simulink model "VisionModel_v16"  (Simulink 7.6)
settings: Solver=FixedStepDiscrete  StartTime=0.0  StopTime=0  RelTol=1e-3
values from neighbouring files (symbols this model uses):
  Buoy_Max_Eccentricity = 1.2    [VisionConstants.m]
  Buoy_Max_Extent = 0.9    [VisionConstants.m]
  Buoy_Min_Eccentricity = 0    [VisionConstants.m]
  Buoy_Min_Extent = 0.1    [VisionConstants.m]
  Down_Camera_Dimensions = [120 160]    [VisionConstants.m]
  Forward_Camera_Dimensions = [160 120]    [VisionConstants.m]
undefined symbols (not defined in the file or in its folder): Forward_Fov, Rec, SDTV
libraries: vipconversions x8, vipgeotforms x6, viptextngfix x6, viptransforms x4, vipanalysis x3
(part 3 of 4)

== matlab function validation_gate/Identify Validation Gate ==
  data: hough_table input double; target_y output double; target_z output double; target_yaw output double; gate_found output double; theta_in input double; rho_in input double; target_height input double; gate_aspect_ratio input double; Forward_Camera_Dimensions input double; Forward_Fov input double; rho_gate output double; theta_gate output double
function [target_y, target_z, target_yaw, gate_found, rho_gate, theta_gate] = validation_gate(hough_table, theta_in, rho_in, target_height, gate_aspect_ratio, Forward_Camera_Dimensions, Forward_Fov)
%#eml



% This function attempts to identfiy the validation gate, and returns
%   targeting information, and a true/false gate_found parameter.
%
% 5-29-11
%
% Input
%
%   target_height = fraction of goal post height to aim AUV at
%   gate_aspect_ratio = used to infer unknown points with little extra
%     processing (height/width of large goalpost-shape)
%
% Output
%
% Notes:
%   The hough_table is destroyed in this function (acceptable if
%     hough_table is not an output)
%   Process:
%     1. Identify primary, relatively "long" lines
%     2. 


%% Initialize
% Only the (max_num_lines) with the most votes will be considered as
%   candidates for the validation gate
max_num_lines = 200;
[rho_length, theta_length] = size(hough_table);
%rows = Forward_Camera_Dimensions(1);
%cols = Forward_Camera_Dimensions(2);
%rows = 120;
%cols = 160;
rows = 160;
cols = 120;


% eps_rho must be at least as big as the gate leg diameter (units of
%   pixels)
eps_rho = .1*max(rows,cols);
% eps_theta is used to distinguish lines as "horizontal" or "vertical";
%   units are radians
eps_theta = 10*pi/180;


% These vectors contain the final three lines that compose the validation gate
rho_gate = zeros(1,3);
theta_gate = zeros(1,3);

% These vectors contain intermediate line information; as lines are
%   eliminated from these vectors, their values are set to zero
rho = zeros(1,max_num_lines);
theta = zeros(1,max_num_lines);





% Identify the most popular max_num_lines lines
i_index = ones(1,max_num_lines);
j_index = ones(1,max_num_lines);

m = 1;
while( m <= max_num_lines )
    
    max_votes = 0;
    for i = 1:rho_length
        for j = 1:theta_length
            if( hough_table(i,j) > max_votes )
                i_index(m) = i;
                j_index(m) = j;
                max_votes = hough_table(i,j);
            end
        end
    end
    
    rho(m) = rho_in(i_index(m));
    theta(m) = theta_in(j_index(m));
    hough_table(i_index(m),j_index(m)) = 0;
    m = m + 1;
    
end


% Effectively generate a small Hough table which contains only values of
%   interest for the validation gate application

rbinv = [0:(2*eps_rho):max(rows, cols)];  % Rho bins for vertical lines
nbinsv = length(rbinv);  % Number of rho bins for vertical lines
ravgv = zeros(1,nbinsv);  % Average rho values for each bin (note that the average value will generally differ slightly than the bin value)
tavgv = zeros(1,nbinsv);  % Average theta values for each bin
vbinv = zeros(1,nbinsv);  % Votes bins for vertical lines

rbinh = [0:(2*eps_rho):max(rows, cols)];
nbinsh = length(rbinh);
ravgh = zeros(1,nbinsh);
tavgh = zeros(1,nbinsh);
vbinh = zeros(1,nbinsh);

% Allow vertical lines along the left side of the image
rbinv(1) = 1;
rbinh(1) = 1;

for i = 1:max_num_lines
    
    % Consider only lines that are either vertical or horizontal, within
    %   tolerance
    condition1 = ( abs(theta(i) - pi/2) <= eps_theta || abs(theta(i) + pi/2) <= eps_theta );  % Horizontal line
    condition2 = ( abs(theta(i) - 0) <= eps_theta );  % Vertical line
    
    if(condition2 && ~( rho(i) == 0 && theta(i) == 0 ))  % Analyze vertical lines (ignore lines exactly along the left side of the image)
        
        for b = 1:nbinsv
            
            % Place each rho value into a bin
            if( abs(rho(i) - rbinv(b)) <= eps_rho )
                ravgv(b) = ravgv(b) + rho(i);
                tavgv(b) = tavgv(b) + theta(i);
                vbinv(b) = vbinv(b) + 1;
                break;
            end
            
        end
        
    elseif(condition1)  % Analyze horizontal lines
        
        if( theta(i) < 0 )
            theta(i) = theta(i) + pi;
            rho(i) = -rho(i);
        end
        
        for b = 1:nbinsh
            
            % Place each rho value into a bin
            if( abs(rho(i) - rbinh(b)) <= eps_rho )
                ravgh(b) = ravgh(b) + rho(i);
                tavgh(b) = tavgh(b) + theta(i);
                vbinh(b) = vbinh(b) + 1;
                break;
            end
            
        end
        
    end
end

% Average the values in ravg and tavg for horizontal and vertical lines
for b = 1:nbinsv
    if( vbinv(b) == 0 )
        ravgv(b) = 0;
        tavgv(b) = 0;
    else
        ravgv(b) = ravgv(b)./vbinv(b);
        tavgv(b) = tavgv(b)./vbinv(b);
    end
end
for b = 1:nbinsh
    if( vbinh(b) == 0 )
        ravgh(b) = 0;
        tavgh(b) = 0;
    else
        ravgh(b) = ravgh(b)./vbinh(b);
        tavgh(b) = tavgh(b)./vbinh(b);
    end
end


%% Extract three lines that fit the criteria for being the validation gate
rmin = 10000;
rmax = -10000;
for b = 1:nbinsv
    
    % Extract the left-most vertical line
    if( ravgv(b) < rmin && ravgv(b) ~= 0 )
        rmin = ravgv(b);
        rho_gate(1) = ravgv(b);
        theta_gate(1) = tavgv(b);
    end
    
    % Extract the right-most vertical line
    if( ravgv(b) > rmax && ravgv(b) ~= 0 )
        rmax = ravgv(b);
        rho_gate(3) = ravgv(b);
        theta_gate(3) = tavgv(b);
    end
    
end

% Check that the distance between the vertical lines is much greater than
%   the minimum expected distance, eps_rho
if( abs(rho_gate(3) - rho_gate(1)) < 2*eps_rho )
    rho_gate(1) = 0;
    rho_gate(3) = 0;
    theta_gate(1) = 0;
    theta_gate(3) = 0;
end

%rmin = 10000;
vmax = 0;
for b = 1:nbinsh
    
    % Extract the horizontal line with the most votes
    if( vbinh(b) > vmax && ravgh(b) ~= 0 )
        vmax = vbinh(b);
        rho_gate(2) = ravgh(b);
        theta_gate(2) = tavgh(b);
    end
    
%    % Extract the horizontal line that is highest up in the image
%    if( ravgh(b) < rmin && ravgh(b) ~= 0 )
%        rmin = ravgh(b);
%        rho_gate(2) = ravgh(b);
%        theta_gate(2) = tavgh(b);
%    end
end


%% Compute targeting information
% Compute intersections
r1 = (  ( rho_gate(1)/cos(theta_gate(1)) ) - ( rho_gate(2)/cos(theta_gate(2)) )  )*(  1/( tan(theta_gate(1)) - tan(theta_gate(2)) )  );
c1 = ( 1/cos(theta_gate(1)) )*( rho_gate(1) - r1*sin(theta_gate(1)) );

r3 = (  ( rho_gate(2)/cos(theta_gate(2)) ) - ( rho_gate(3)/cos(theta_gate(3)) )  )*(  1/( tan(theta_gate(2)) - tan(theta_gate(3)) )  );
c3 = ( 1/cos(theta_gate(2)) )*( rho_gate(2) - r3*sin(theta_gate(2)) );

r2 = (r1 + r3)/2;
c2 = (c1 + c3)/2;

% Compute gate width
w = sqrt( (r3 - r1)^2 + (c3 - c1)^2 );

% Form unit vector pointing downward, parallel to gate posts
tavg = ( theta_gate(1) + (theta_gate(2) - pi/2) + theta_gate(3) )/3;
u = [1 tan(tavg)];
u = u./norm(u);

% Compute target location
th = target_height*gate_aspect_ratio*w;
r_t = r2 + th*u(1);
c_t = c2 + th*u(2);

% Determine if a gate is present (very simple, potentially inaccurate)
if( sum( (rho_gate == 0) + (theta_gate == 0) ) > 0 )
    
    gate_found = 0;
    target_z = 0;
    target_y = 0;
    target_yaw = 0;
    
else
    
    gate_found = 1;
    
    % Transform target r, c to global coordinate system
    target_z = r_t - floor(rows/2);
    target_y = c_t - floor(cols/2);
    target_yaw = Forward_Fov*(target_y/cols);
    
end


return

== matlab function validation_gate/If Action Subsystem/Transform Coordinates3 ==
  data: which_camera input double; x_in input double; y_in input double; z_in input double; Camera_Dimensions input double; points output double
function points = transform_G2L(which_camera, x_in, y_in, z_in, Camera_Dimensions)
% This function, "transform Global to Local coordinates," transforms
%   global coordinates that are sent to the controller into local
%   coordinates that can be displayed over images.
%
% 5-29-11
%
% Input
%   x_in, y_in, z_in = vectors of points in global (vehicle-centered)
%     coordinate system
%   bw_image_in = a 2-D array of pixel values (used only to extract image
%     size)
%   which_camera = selects which camera for relative coordinates
%                = 0 -> Forward camera
%                = 1 -> Down camera
%
% Output
%   r_out, c_out = row, column pairs in local coordinate system

rows = Camera_Dimensions(1);
cols = Camera_Dimensions(2);
if( which_camera == 0 )
    points = [z_in + floor(rows/2);
              y_in + floor(cols/2)];
else
    points = [floor(rows/2) - x_in;
              y_in + floor(cols/2)];
end


return

== matlab function L_detector/If Action Subsystem/Transform Coordinates3 ==
  data: which_camera input double; x_in input double; y_in input double; z_in input double; Camera_Dimensions input double; points output double
function points = transform_G2L(which_camera, x_in, y_in, z_in, Camera_Dimensions)
% This function, "transform Global to Local coordinates," transforms
%   global coordinates that are sent to the controller into local
%   coordinates that can be displayed over images.
%
% 5-29-11
%
% Input
%   x_in, y_in, z_in = vectors of points in global (vehicle-centered)
%     coordinate system
%   bw_image_in = a 2-D array of pixel values (used only to extract image
%     size)
%   which_camera = selects which camera for relative coordinates
%                = 0 -> Forward camera
%                = 1 -> Down camera
%
% Output
%   r_out, c_out = row, column pairs in local coordinate system

rows = Camera_Dimensions(1);
cols = Camera_Dimensions(2);
if( which_camera == 0 )
    points = [z_in + floor(rows/2);
              y_in + floor(cols/2)];
else
    points = [floor(rows/2) - x_in;
              y_in + floor(cols/2)];
end


return

== matlab function Blob_Analysis1/Blob Extraction ==
  data: LabelMatrix input double; num_colors input double; ref_colors input double; blob_hues output double; blob_area output double; blob_centroids output double; blob_bbox output double; blob_major_axis output double; blob_minor_axis output double; blob_orientation output double; blob_eccentricity output double; blob_extent output double; blob_count output double; blob_color output double; bw_image output double; ColorFilter_in input double
function [blob_hues, blob_area, blob_centroids, blob_bbox, blob_major_axis, blob_minor_axis, blob_orientation, blob_eccentricity, blob_extent, blob_count, blob_color, bw_image] = GetBlobInfo(LabelMatrix, num_colors, ref_colors, ColorFilter_in)
% This function calculates blob information for each color component after
%   iterative segmentation


% Output
%   blob_color = 1xN vector of color indices (global color scheme)


% Initialize


%{
a_range =[0     0     0    25   127    70    50;
     0     0     0   127   -18   -40   -82];


b_range =[0     0     0     0    30   -13   -40;
     0     0     0    56   -10    30     9];
%}

%ColorFilter = ColorFilter_in;



cf = [0 1 0 0 0 0 0;
0     0     0    25   127    70    50;
0     0     0   127   -18   -40   -82;
0     0     0     0    30   -13   -40;
0     0     0    56   -10    30     9];

ColorFilter = ColorFilter_in(:,1);
a_range = cf(2:3,:);
b_range = cf(4:5,:);

max_num_blobs = 50;
min_blob_area = 5;

[rows, cols] = size(LabelMatrix);
image_area = rows*cols;
LogicMatrix = false(rows,cols);
bw_image = zeros(rows,cols);

blob_hues = zeros(3,max_num_blobs);
blob_area = -1.*ones(1,max_num_blobs);
blob_bbox = zeros(4,max_num_blobs);
blob_major_axis = zeros(1,max_num_blobs);
blob_minor_axis = zeros(1,max_num_blobs);
blob_centroids = zeros(2,max_num_blobs);
blob_eccentricity = zeros(1,max_num_blobs);
blob_extent = zeros(1,max_num_blobs);
blob_orientation = zeros(1,max_num_blobs);
blob_count = 0;

blob_color = zeros(1,max_num_blobs);

max_num_col_filter = length(ColorFilter);
num_col_filter = sum(ColorFilter);

area_thresh = .1;


% Determine L_white and L_black as needed
find_white = 0;
find_black = 0;
L_white = 101;
L_black = -1;
color_areas = zeros(1,size(ref_colors,1));

if(ColorFilter(1) + ColorFilter(2) > 0)
    for row = 1:rows
        for col = 1:cols
            color_areas(LabelMatrix(row,col)) = color_areas(LabelMatrix(row,col)) + 1;
        end
    end
end

if(ColorFilter(1) == 1)
    
    % Determine the brightest colors, but allow a maximum area
    %   ratio of the image to be "white"
    find_white = 1;
    
    positive_area = 0;
    for n = 1:num_colors
        
        maxL = -1;
        k_max = -1;
        for k = 1:num_colors
            L = ref_colors(k,1);
            if(L > maxL && L < L_white)
                maxL = L;
                k_max = k;
            end
        end
        
        positive_area = positive_area + color_areas(k_max);
        if(positive_area/image_area >= area_thresh && n > 1)
            break;
        end
        
        L_white = maxL;
        
    end
end

if(ColorFilter(2) == 1)
    
    % Determine the darkest colors, but allow a maximum area
    %   ratio of the image to be "black"
    find_black = 1;
    
    for row = 1:rows
        for col = 1:cols
            color_areas(LabelMatrix(row,col)) = color_areas(LabelMatrix(row,col)) + 1;
        end
    end
    
    positive_area = 0;
    for n = 1:num_colors
        
        minL = 101;
        k_min = -1;
        for k = 1:num_colors
            L = ref_colors(k,1);
            if(L < minL && L > L_black)
                minL = L;
                k_min = k;
            end
        end
        
        positive_area = positive_area + color_areas(k_min);
        if(positive_area/image_area >= area_thresh && n > 1)
            break;
        end
        
        L_black = minL;
        
    end
end


% Input hblob, a matrix containing [Area, blob_centroids, Eccentricity] for each
% identified blob
persistent hblob
if isempty(hblob)
    hblob = video.BlobAnalysis('AreaOutputPort',true,'CentroidOutputPort',true,...
        'BoundingBoxOutputPort',true,'MajorAxisLengthOutputPort',true,'MinorAxisLengthOutputPort',true,...
        'OrientationOutputPort',true,...
        'EccentricityOutputPort',true,'ExtentOutputPort',true,'NumBlobsOutputPort',true,...
        'MinimumBlobAreaSource','Property','MinimumBlobArea', min_blob_area);
end


% Calculate geometric information about the blobs
%
% LogicMatrix is a binary version of LabelMatrix, with ones at all
%   locations for which color values are k, and zeros everywhere else
%
% Explanation
%   condition1 == 1 causes the k'th color to be analyzed by blob analysis,
%     as well as be included in the black-and-white image
%   condition1 == 0 disallows both of these items and simply ignores color
%     k
%   condition0 == 1 ensures that condition1 is true for all k
%   condition0 == 0 enforces a filter which allows only the colors
%     specified in the ColorFilter vector
condition0 = (num_col_filter == 0);
current_color = 0;
for k = 1:num_colors
    
    % Decide whether or not to perform blob analysis
    condition1 = 0;
    if(condition0)
        condition1 = 1;
    else
        a = ref_colors(k, 2);
        b = ref_colors(k, 3);
        for i = 1:max_num_col_filter
            
            % Skip colors that have not been specified
            if(ColorFilter(i) == 0)
                continue;
            end
            
            if( find_white == 1 && ref_colors(k,1) >= L_white)  % Handle "white" differently than other colors
                condition1 = 1;
                current_color = 1;
                break;
            elseif( find_black == 1 && ref_colors(k,1) <= L_black)  % Handle "black" differently than other colors
                condition1 = 1;
                current_color = 2;
                break;
            elseif( a >= a_range(1,i) && a <= a_range(2,i) && b >= b_range(1,i) && b <= b_range(2,i) )
                condition1 = 1;
                current_color = i;
                break;
            end
            
        end
    end
    
    % Blob analysis
    if( condition1 == 1 )
        
        for i = 1:rows
            for j = 1:cols
                if(LabelMatrix(i,j) ~= k)
                    LogicMatrix(i,j) = false;
                else
                    LogicMatrix(i,j) = true;
                    bw_image(i,j) = 1;
                end
            end
        end

        [TArea,TCentroid,TBBox,TMajorAxis,TMinorAxis,TOrientation,TEccent,TExtent,TNumBlobs] = step(hblob,LogicMatrix);

        for i = 1:TNumBlobs
            if(blob_count + TNumBlobs <= max_num_blobs)

                blob_centroids(1,blob_count+i) = TCentroid(1,i);
                blob_centroids(2,blob_count+i) = TCentroid(2,i);

                ii = round(blob_centroids(1,blob_count+i));
                jj = round(blob_centroids(2,blob_count+i));

                blob_hues(1,blob_count+i) = ref_colors( LabelMatrix(ii,jj), 1 );
                blob_hues(2,blob_count+i) = ref_colors( LabelMatrix(ii,jj), 2 );
                blob_hues(3,blob_count+i) = ref_colors( LabelMatrix(ii,jj), 3 );

                blob_area(blob_count+i) = TArea(i);
                blob_bbox(blob_count+i) = TBBox(i);
                blob_major_axis(blob_count+i) = TMajorAxis(i);
                blob_minor_axis(blob_count+i) = TMinorAxis(i);
                blob_eccentricity(blob_count+i) = TEccent(i);
                blob_extent(blob_count+i) = TExtent(i);
                blob_orientation(blob_count+i) = TOrientation(i);
                
                blob_color(blob_count+i) = current_color;

            end
        end

        blob_count = blob_count + double(TNumBlobs);

    end
    
end


return

== matlab function Blob_Analysis1/IterativeSegmentation/Low Pass Filter/Low Pass Filter ==
  data: I input double; Iout output double
function Iout = GaussianBlurr(I)
% This function calculates the gaussian blur of an intensity image

sigma = sqrt(2);

Grows = 3;    % Gaussian matrix rows
Gcols = 3;    % Gaussian matrix columns

[Irows Icols] = size(I);

Iout = double(zeros(Irows,Icols));

Trows = Irows - Grows + 1;
Tcols = Icols - Gcols + 1;
Itemp = double(zeros(Trows,Tcols));

G = zeros(Grows,Gcols);

FirstRow = ceil(-Grows/2);
LastRow = floor(Grows/2);
FirstCol = ceil(-Gcols/2);
LastCol = floor(Gcols/2);
Gsum = 0;
for i=FirstRow:LastRow
    for j = FirstCol:LastCol
        G(i-FirstRow+1,j-FirstCol+1) = exp(-(j*j+i*i)/(2*sigma*sigma));
        Gsum = Gsum + G(i-FirstRow+1,j-FirstCol+1);
    end
end

G = G./Gsum;

Itemp = conv2(double(I),double(G),'valid');

% reflect boundaries to keep image the same size
% top
Iout((1:LastRow),(LastCol+1:Icols-LastCol)) = Itemp((1:LastRow),(1:Tcols));
% bottom
Iout((Irows-LastRow+1:Irows),(LastCol+1:Icols-LastCol)) = Itemp((Trows-LastRow+1:Trows),(1:Tcols));
% left
Iout((1+LastRow:Irows-LastRow),(1:LastCol)) = Itemp((1:Trows),(1:LastCol));
% right
Iout((1+LastRow:Irows-LastRow),(Icols-LastCol+1:Icols)) = Itemp((1:Trows),(Tcols-LastCol+1:Tcols));
% center
Iout((1+LastRow:Irows-LastRow),(1+LastCol:Icols-LastCol)) = Itemp;
% top left corner
Iout(1:LastRow,1:LastCol) = Itemp(1:LastRow,1:LastCol);
% top right corner
Iout(1:LastRow,Icols-LastCol:Icols) = Itemp(1:LastRow,Tcols-LastCol:Tcols);
% bottom left corner
Iout(Irows-LastRow:Irows,1:LastCol) = Itemp(Trows-LastRow:Trows,1:LastCol);
% bottom right corner
Iout(Irows-LastRow:Irows,Icols-LastCol:Icols) = Itemp(Trows-LastRow:Trows,Tcols-LastCol:Tcols);

return

== matlab function Blob_Analysis1/IterativeSegmentation/Low Pass Filter/Low Pass Filter1 ==
  data: I input double; Iout output double
function Iout = GaussianBlurr(I)
% This function calculates the gaussian blur of an intensity image

sigma = sqrt(2);

Grows = 3;    % Gaussian matrix rows
Gcols = 3;    % Gaussian matrix columns

[Irows Icols] = size(I);

Iout = double(zeros(Irows,Icols));

Trows = Irows - Grows + 1;
Tcols = Icols - Gcols + 1;
Itemp = double(zeros(Trows,Tcols));

G = zeros(Grows,Gcols);

FirstRow = ceil(-Grows/2);
LastRow = floor(Grows/2);
FirstCol = ceil(-Gcols/2);
LastCol = floor(Gcols/2);
Gsum = 0;
for i=FirstRow:LastRow
    for j = FirstCol:LastCol
        G(i-FirstRow+1,j-FirstCol+1) = exp(-(j*j+i*i)/(2*sigma*sigma));
        Gsum = Gsum + G(i-FirstRow+1,j-FirstCol+1);
    end
end

G = G./Gsum;

Itemp = conv2(double(I),double(G),'valid');

% reflect boundaries to keep image the same size
% top
Iout((1:LastRow),(LastCol+1:Icols-LastCol)) = Itemp((1:LastRow),(1:Tcols));
% bottom
Iout((Irows-LastRow+1:Irows),(LastCol+1:Icols-LastCol)) = Itemp((Trows-LastRow+1:Trows),(1:Tcols));
% left
Iout((1+LastRow:Irows-LastRow),(1:LastCol)) = Itemp((1:Trows),(1:LastCol));
% right
Iout((1+LastRow:Irows-LastRow),(Icols-LastCol+1:Icols)) = Itemp((1:Trows),(Tcols-LastCol+1:Tcols));
% center
Iout((1+LastRow:Irows-LastRow),(1+LastCol:Icols-LastCol)) = Itemp;
% top left corner
Iout(1:LastRow,1:LastCol) = Itemp(1:LastRow,1:LastCol);
% top right corner
Iout(1:LastRow,Icols-LastCol:Icols) = Itemp(1:LastRow,Tcols-LastCol:Tcols);
% bottom left corner
Iout(Irows-LastRow:Irows,1:LastCol) = Itemp(Trows-LastRow:Trows,1:LastCol);
% bottom right corner
Iout(Irows-LastRow:Irows,Icols-LastCol:Icols) = Itemp(Trows-LastRow:Trows,Tcols-LastCol:Tcols);

return

== matlab function Blob_Analysis1/IterativeSegmentation/Low Pass Filter/Low Pass Filter2 ==
  data: I input double; Iout output double
function Iout = GaussianBlurr(I)
% This function calculates the gaussian blur of an intensity image

sigma = sqrt(2);

Grows = 3;    % Gaussian matrix rows
Gcols = 3;    % Gaussian matrix columns

[Irows Icols] = size(I);

Iout = double(zeros(Irows,Icols));

Trows = Irows - Grows + 1;
Tcols = Icols - Gcols + 1;
Itemp = double(zeros(Trows,Tcols));

G = zeros(Grows,Gcols);

FirstRow = ceil(-Grows/2);
LastRow = floor(Grows/2);
FirstCol = ceil(-Gcols/2);
LastCol = floor(Gcols/2);
Gsum = 0;
for i=FirstRow:LastRow
    for j = FirstCol:LastCol
        G(i-FirstRow+1,j-FirstCol+1) = exp(-(j*j+i*i)/(2*sigma*sigma));
        Gsum = Gsum + G(i-FirstRow+1,j-FirstCol+1);
    end
end

G = G./Gsum;

Itemp = conv2(double(I),double(G),'valid');

% reflect boundaries to keep image the same size
% top
Iout((1:LastRow),(LastCol+1:Icols-LastCol)) = Itemp((1:LastRow),(1:Tcols));
% bottom
Iout((Irows-LastRow+1:Irows),(LastCol+1:Icols-LastCol)) = Itemp((Trows-LastRow+1:Trows),(1:Tcols));
% left
Iout((1+LastRow:Irows-LastRow),(1:LastCol)) = Itemp((1:Trows),(1:LastCol));
% right
Iout((1+LastRow:Irows-LastRow),(Icols-LastCol+1:Icols)) = Itemp((1:Trows),(Tcols-LastCol+1:Tcols));
% center
Iout((1+LastRow:Irows-LastRow),(1+LastCol:Icols-LastCol)) = Itemp;
% top left corner
Iout(1:LastRow,1:LastCol) = Itemp(1:LastRow,1:LastCol);
% top right corner
Iout(1:LastRow,Icols-LastCol:Icols) = Itemp(1:LastRow,Tcols-LastCol:Tcols);
% bottom left corner
Iout(Irows-LastRow:Irows,1:LastCol) = Itemp(Trows-LastRow:Trows,1:LastCol);
% bottom right corner
Iout(Irows-LastRow:Irows,Icols-LastCol:Icols) = Itemp(Trows-LastRow:Trows,Tcols-LastCol:Tcols);

return

== matlab function Blob_Analysis1/IterativeSegmentation/Segmentation/LabSegmentation ==
  data: L input double; LabelMatrix output double; a input double; b input double; ref_colors input double; num_colors input double
function LabelMatrix  = LabSegmentation(L,a,b,ref_colors,num_colors)
% This function generates the label matrix

[rows cols] = size(L);
LabelMatrix = zeros(rows,cols);

for i = 1:rows
    for j = 1:cols
        min_dist = 1000;
        index = 1;
        for k = 1:num_colors
            dist = sqrt((ref_colors(k,1) - L(i,j))^2 + (ref_colors(k,2) - a(i,j))^2 + (ref_colors(k,3) - b(i,j))^2);
            if(dist < min_dist)
                min_dist = double(dist);
                index = k;
            end
        end
        LabelMatrix(i,j) = index;
    end
end


return

== matlab function Blob_Analysis1/IterativeSegmentation/Segmentation/Reference Color Selection ==
  data: L input double; ref_colors output double; a input double; b input double; num_colors output double; Dist_Thresh input double
function [ref_colors, num_colors] = Segmentation(L,a,b,Dist_Thresh)
% This function tries segmentation by adding new reference colors everytime
% a pixel is found with a distance greater than a certain amount from
% every other reference color

[rows cols] = size(L);

Dist_Threshold = Dist_Thresh;% L = 0 to 100, a = -100 to 100, b = -100 to 100
                    % max dist = 300 -> 60/300 is 20%
x = 1;  % coefficients determining distance calculation
y = 1.5;
z = 1.5;

max_num_colors = 50;
ref_colors = zeros(max_num_colors,3);   % At most 50 different reference colors
LabelMatrix = zeros(rows,cols);
num_colors = 1;

center_row = floor(rows/2);
center_col = floor(cols/2);

% Define first reference color to be colr
ref_colors(1,:) = [L(center_row,center_col) a(center_row,center_col) b(center_row,center_col)];

flag = 0;
i = 1;
j = 1;
while(i <= rows)        % perform initial segmentation
    while(i <= rows && flag == 0)
        while(j <= cols && flag == 0)
            k = 1;
            min_dist = 1000;
            index = 1;
            while(k <= num_colors)
                dist = sqrt(x*(ref_colors(k,1) - L(i,j))^2 + y*(ref_colors(k,2) - a(i,j))^2 + z*(ref_colors(k,3) - b(i,j))^2);
                if(min_dist > dist)
                    min_dist = double(dist);
                    index = k;
                end
                k = k + 1;
            end
            if(j == 117)
                cow = 1;
            end
            if(min_dist > Dist_Threshold && num_colors < max_num_colors)
                ref_colors(num_colors+1,:) = [L(i,j) a(i,j) b(i,j)];
                num_colors = num_colors + 1;
                flag = 1;
                i = 0;
                j = 0;
            else
                LabelMatrix(i,j) = index;
            end
            j = j + 1;
        end
        j = 1;
        i = i + 1;
    end
    flag = 0;
end

% Go through image once more to get more accurate values for the different regions
ref_color_L_avg = zeros(50,1);
ref_color_a_avg = zeros(50,1);
ref_color_b_avg = zeros(50,1);
color_count = zeros(50,1);
for i = 1:rows
    for j = 1:cols
        index = LabelMatrix(i,j);
        ref_color_L_avg(index) = ref_color_L_avg(index) + L(i,j);
        ref_color_a_avg(index) = ref_color_a_avg(index) + a(i,j);
        ref_color_b_avg(index) = ref_color_b_avg(index) + b(i,j);
        color_count(index) = color_count(index) + 1;
    end
end
ref_color_L_avg = ref_color_L_avg ./ color_count;
ref_color_a_avg = ref_color_a_avg ./ color_count;
ref_color_b_avg = ref_color_b_avg ./ color_count;

for i = 1:num_colors
    ref_colors(i,1) = ref_color_L_avg(i);
    ref_colors(i,2) = ref_color_a_avg(i);
    ref_colors(i,3) = ref_color_b_avg(i);
end

return

== matlab function Blob_Analysis1/Segmented Image/Display Image ==
  data: LabelMatrix input double; ref_colors input double; L output double; a output double; b output double
function [L, a, b] = Display_Image(LabelMatrix, ref_colors)


% Initialize
[rows,cols] = size(LabelMatrix);
L = zeros(rows,cols);
a = zeros(rows,cols);
b = zeros(rows,cols);


% Allow only colors in specified range
for r = 1:rows
    for c = 1:cols
        
        L(r,c) = ref_colors(LabelMatrix(r,c), 1);
        a(r,c) = ref_colors(LabelMatrix(r,c), 2);
        b(r,c) = ref_colors(LabelMatrix(r,c), 3);
        
    end
end


return

== matlab function path_detector/Identify Path Elements ==
  data: hough_table input double; theta_in input double; rho_in input double; blob_count input double; blob_area input double; blob_centroids input double; blob_orientation input double; Down_Camera_Dimensions input double; theta output double; rho output double; path_headings output double; path_found output double; rho_out output double; theta_out output double; orientation output double
function [theta, rho, path_headings, path_found, rho_out, theta_out, orientation] = path_detection(hough_table, theta_in, rho_in, blob_count, blob_area, blob_centroids, blob_orientation, Down_Camera_Dimensions)
%#eml

% This function attempts to identfiy path elements, and returns lines,
%   information about the paths that are present, and a true/false
%   path_found parameter.
%
% 5-30-11
%
% Input
%
% Output
%  path_headings = vector of path orientations in terms of headings
%    relative to the auv (degrees)
%  rho, theta = vectors containing lines determined by Hough Transform,
%    ordered by number of votes
%
% Notes:
%   The hough_table is destroyed in this function (acceptable if
%     hough_table is not an output)
%   blob_orientation is destroyed


% Initialize
max_num_lines = 200;  % Considers this many popular lines as candidates
max_num_paths = 3;

[rho_length, theta_length] = size(hough_table);
rows = Down_Camera_Dimensions(1);
cols = Down_Camera_Dimensions(2);
image_area = rows*cols;

rho_tol = .1*max(rows,cols);  % Tolerance within which two lines are coincident
theta_tol = 10*pi/180;  % Tolerence within which two slopes are equal (radians)
area_thresh = 0.8;  % Ratio of blob area to image area considered to imply the blob is actually background noise

rho = zeros(1,max_num_lines);
theta = zeros(1,max_num_lines);
theta_hold = zeros(1,max_num_lines);  % theta_hold is a copy of theta which gets destroyed

rho_out = zeros(1,max_num_lines);
theta_out = zeros(1,max_num_lines);

path_headings = 1000.*ones(1,max_num_paths);  % 1000 is an invalid angle
path_locations = zeros(2,max_num_paths);
path_found = 0;
%path_found_vector = zeros(1,max_num_paths);


% Identify the most likely max_num_lines lines
for( m = 1:max_num_lines )
    
    max_votes = 0;
    i_index = 1;
    j_index = 1;
    for i = 1:rho_length
        for j = 1:theta_length
            if( hough_table(i,j) > max_votes )
                i_index = i;
                j_index = j;
                max_votes = hough_table(i,j);
            end
        end
    end
    
    if(max_votes == 0)
        break;
    end
    
    rho(m) = rho_in(i_index);
    theta(m) = theta_in(j_index);
    theta_hold(m) = theta_in(j_index);
    hough_table(i_index,j_index) = 0;
    
end    


% Correct orientations to vehicle coordinates
for j = 1:blob_count
    % theta_hold:
    %   -is between [-pi/2, +pi/2]
    % blob_orientation:
    %   -is potentially outside this range
    %   -needs to be corrected by pi/2 to get relative heading
%    blob_orientation(j) = (pi/2) - blob_orientation(j);

    blob_orientation(j) = mod(pi - blob_orientation(j), pi) - pi/2;
%    if(blob_orientation(j) > pi/2)
%        blob_orientation(j) = blob_orientation(j) - pi;
%    elseif(blob_orientation(j) < -pi/2)
%        blob_orientation(j) = blob_orientation(j) + pi;
%    end
end


% Compare most popular lines with blob orientations
c = 1;
for p = 1:max_num_paths
    
    found = 0;
    for i = 1:max_num_lines
        for j = 1:blob_count
            
            % Search for a match between one blob and one line
            if( abs(theta_hold(i) - blob_orientation(j)) <= theta_tol  &&  blob_area(j)/image_area <= area_thresh  &&  (theta_hold(i) ~= 1000 && blob_orientation(j) ~= 1000) )
                path_headings(p) = theta_hold(i);
%                path_found_vector(p) = 
                path_locations(1,p) = blob_centroids(1,j);
                path_locations(2,p) = blob_centroids(2,j);
                
                
                
                %
                rho_out(c) = rho(i);
                theta_out(c) = theta(i);
                c = c + 1;
                %/
                
                
                theta_hold(i) = 1000;  % Invalid angle; do not want this line to be selected again
                blob_orientation(j) = 1000;
                found = 1;
                break;
            end
            
        end
        
        if(found == 1)
            break;
        end
    end
    
end


% Order path_headings to reflect actual path locations (left to right in
%   image)
value = Down_Camera_Dimensions(2).*ones(1,max_num_paths);
j_index = ones(1,max_num_paths);
found = zeros(1,max_num_paths);

for p = 1:max_num_paths
    for j = 1:max_num_paths
        if(path_locations(2,j) < value(p) && found(j) == 0)
            value(p) = path_locations(2,j);
            j_index(p) = j;
        end
    end
    found(j_index(p)) = 1;
end

matr = [path_headings; path_locations];
for p = 1:max_num_paths
    path_headings(p) = matr(1,j_index(p));
    path_locations(1,p) = matr(2,j_index(p));
    path_locations(2,p) = matr(3,j_index(p));
end


















% old code \/ \/

% Determine which way the 'Y' shape is pointing
%path_headings = sort(path_headings, 2, 'ascend');
%heading_diff = abs([ path_headings(2) - path_headings(1), path_headings(3) - path_headings(2), path_headings(1) - path_headings(3)]);
%if(heading_diff(1) < heading_diff(2) && heading_diff(1) < heading_diff(3))
%    y_heading = path_headings(3);
%elseif(heading_diff(2) < heading_diff(1) && heading_diff(2) < heading_diff(3))
%    y_heading = path_headings(1);
%elseif(heading_diff(3) < heading_diff(1) && heading_diff(3) < heading_diff(2))
%    y_heading = path_headings(2);
%else
%    y_heading = 0;
%end




% Determine a good approximation of the median lines (ignore effectively
%   duplicate lines)
%{
rho(1) = rho(1);
theta(1) = theta(1);

m = 2;
for i = 2:max_num_lines
    
    % If rho, theta do not match within tolerance, then store as the next
    %   line
    if( abs(rho(i) - rho(i-1)) >= 30 )
        rho_out(m) = rho(i);
        theta_out(m) = theta(i);
        m = m + 1;
        if( m > 3 )
            break;
        end
    end
    
end




% Select the most popular lines assuming that they correspond to the path
%   edges
%}




theta = theta_hold;
orientation = blob_orientation;

return

== matlab function path_detector/Identify Path Elements1 ==
  data: path_headings input double; path_found input double; target_x output double; target_y output double; target_yaw output double; path_state output double; which_path input double
function [target_x, target_y, target_yaw, path_state] =  choose_path(path_headings, path_found, which_path)
%#eml

% Input
%   which_path = indicates which direction to take; left (1) right (2) or
%     straight (0)

% Return the relative heading of the path element pointing "left" or
%   "right"
if(which_path == 1)
    % Take leftmost path
    target_yaw = 1000;
    for n = 1:length(path_headings)
        if(path_headings(n) < target_yaw && path_headings(n) ~= 1000)
            target_yaw = path_headings(n);
        end
    end
    target_yaw = target_yaw*180/pi;
%    target_yaw = min(path_headings)*180/pi;

elseif(which_path == 2)
    % Take rightmost path
    target_yaw = -1000;
    for n = 1:length(path_headings)
        if(path_headings(n) > target_yaw && path_headings(n) ~= 1000)
            target_yaw = path_headings(n);
        end
    end
    target_yaw = target_yaw*180/pi;
%    target_yaw = max(path_headings)*180/pi;

else
    % Continue straight
    target_yaw = 0;
end

target_x = 0;
target_y = 0;
path_state = 0;

return

== matlab function path_detector/If Action Subsystem/Transform Coordinates3 ==
  data: which_camera input double; x_in input double; y_in input double; z_in input double; Camera_Dimensions input double; points output double
function points = transform_G2L(which_camera, x_in, y_in, z_in, Camera_Dimensions)
% This function, "transform Global to Local coordinates," transforms
%   global coordinates that are sent to the controller into local
%   coordinates that can be displayed over images.
%
% 5-29-11
%
% Input
%   x_in, y_in, z_in = vectors of points in global (vehicle-centered)
%     coordinate system
%   bw_image_in = a 2-D array of pixel values (used only to extract image
%     size)
%   which_camera = selects which camera for relative coordinates
%                = 0 -> Forward camera
%                = 1 -> Down camera
%
% Output
%   r_out, c_out = row, column pairs in local coordinate system

rows = Camera_Dimensions(1);
cols = Camera_Dimensions(2);
if( which_camera == 0 )
    points = [z_in + floor(rows/2);
              y_in + floor(cols/2)];
else
    points = [floor(rows/2) - x_in;
              y_in + floor(cols/2)];
end


return

== matlab function Blob Extraction1 ==
  data: ColorFilter_in input double; a_range input double; ColorFilter_out output double; b_range input double
function ColorFilter_out = concatRanges(ColorFilter_in, a_range, b_range)

% 7-15-11
% This function exists solely to solve an untraceable parsing error in the
%   Simulink compiler. This error has to do with having two Blob Analysis
%   function blocks in the same model.

ColorFilter_out = [ColorFilter_in'; a_range; b_range];

== matlab function Blob Extraction2 ==
  data: ColorFilter_in input double; a_range input double; ColorFilter_out output double; b_range input double
function ColorFilter_out = concatRangesT(ColorFilter_in, a_range, b_range)

% 7-15-11
% This function exists solely to solve an untraceable parsing error in the
%   Simulink compiler. This error has to do with having two Blob Analysis
%   function blocks in the same model.

ColorFilter_out = [ColorFilter_in];
%ColorFilter_out = [ColorFilter_in, a_range', b_range'];

== matlab function Blob_Analysis/Blob Extraction ==
  data: LabelMatrix input double; num_colors input double; ref_colors input double; ColorFilter input double; a_range input double; b_range input double; blob_hues output double; blob_area output double; blob_centroids output double; blob_bbox output double; blob_major_axis output double; blob_minor_axis output double; blob_orientation output double; blob_eccentricity output double; blob_extent output double; blob_count output double; blob_color output double; bw_image output double
function [blob_hues, blob_area, blob_centroids, blob_bbox, blob_major_axis, blob_minor_axis, blob_orientation, blob_eccentricity, blob_extent, blob_count, blob_color, bw_image] = GetBlobInfo(LabelMatrix, num_colors, ref_colors, ColorFilter, a_range, b_range)
% This function calculates blob information for each color component after
%   iterative segmentation


% Output
%   blob_color = 1xN vector of color indices (global color scheme)


% Initialize
max_num_blobs = 50;
min_blob_area = 5;

[rows, cols] = size(LabelMatrix);
image_area = rows*cols;
LogicMatrix = false(rows,cols);
bw_image = zeros(rows,cols);

blob_hues = zeros(3,max_num_blobs);
blob_area = -1.*ones(1,max_num_blobs);
blob_bbox = zeros(4,max_num_blobs);
blob_major_axis = zeros(1,max_num_blobs);
blob_minor_axis = zeros(1,max_num_blobs);
blob_centroids = zeros(2,max_num_blobs);
blob_eccentricity = zeros(1,max_num_blobs);
blob_extent = zeros(1,max_num_blobs);
blob_orientation = zeros(1,max_num_blobs);
blob_count = 0;

blob_color = zeros(1,max_num_blobs);

max_num_col_filter = length(ColorFilter);
num_col_filter = sum(ColorFilter);

area_thresh = .1;


% Determine L_white and L_black as needed
find_white = 0;
find_black = 0;
L_white = 101;
L_black = -1;
color_areas = zeros(1,size(ref_colors,1));

if(ColorFilter(1) + ColorFilter(2) > 0)
    for row = 1:rows
        for col = 1:cols
            color_areas(LabelMatrix(row,col)) = color_areas(LabelMatrix(row,col)) + 1;
        end
    end
end

if(ColorFilter(1) == 1)
    
    % Determine the brightest colors, but allow a maximum area
    %   ratio of the image to be "white"
    find_white = 1;
    
    positive_area = 0;
    for n = 1:num_colors
        
        maxL = -1;
        k_max = -1;
        for k = 1:num_colors
            L = ref_colors(k,1);
            if(L > maxL && L < L_white)
                maxL = L;
                k_max = k;
            end
        end
        
        positive_area = positive_area + color_areas(k_max);
        if(positive_area/image_area >= area_thresh && n > 1)
            break;
        end
        
        L_white = maxL;
        
    end
end

if(ColorFilter(2) == 1)
    
    % Determine the darkest colors, but allow a maximum area
    %   ratio of the image to be "black"
    find_black = 1;
    
    for row = 1:rows
        for col = 1:cols
            color_areas(LabelMatrix(row,col)) = color_areas(LabelMatrix(row,col)) + 1;
        end
    end
    
    positive_area = 0;
    for n = 1:num_colors
        
        minL = 101;
        k_min = -1;
        for k = 1:num_colors
            L = ref_colors(k,1);
            if(L < minL && L > L_black)
                minL = L;
                k_min = k;
            end
        end
        
        positive_area = positive_area + color_areas(k_min);
        if(positive_area/image_area >= area_thresh && n > 1)
            break;
        end
        
        L_black = minL;
        
    end
end


% Input hblob, a matrix containing [Area, blob_centroids, Eccentricity] for each
% identified blob
persistent hblob
if isempty(hblob)
    hblob = video.BlobAnalysis('AreaOutputPort',true,'CentroidOutputPort',true,...
        'BoundingBoxOutputPort',true,'MajorAxisLengthOutputPort',true,'MinorAxisLengthOutputPort',true,...
        'OrientationOutputPort',true,...
        'EccentricityOutputPort',true,'ExtentOutputPort',true,'NumBlobsOutputPort',true,...
        'MinimumBlobAreaSource','Property','MinimumBlobArea', min_blob_area);
end


% Calculate geometric information about the blobs
%
% LogicMatrix is a binary version of LabelMatrix, with ones at all
%   locations for which color values are k, and zeros everywhere else
%
% Explanation
%   condition1 == 1 causes the k'th color to be analyzed by blob analysis,
%     as well as be included in the black-and-white image
%   condition1 == 0 disallows both of these items and simply ignores color
%     k
%   condition0 == 1 ensures that condition1 is true for all k
%   condition0 == 0 enforces a filter which allows only the colors
%     specified in the ColorFilter vector
condition0 = (num_col_filter == 0);
current_color = 0;
for k = 1:num_colors
    
    % Decide whether or not to perform blob analysis
    condition1 = 0;
    if(condition0)
        condition1 = 1;
    else
        a = ref_colors(k, 2);
        b = ref_colors(k, 3);
        for i = 1:max_num_col_filter
            
            % Skip colors that have not been specified
            if(ColorFilter(i) == 0)
                continue;
            end
            
            if( find_white == 1 && ref_colors(k,1) >= L_white)  % Handle "white" differently than other colors
                condition1 = 1;
                current_color = 1;
                break;
            elseif( find_black == 1 && ref_colors(k,1) <= L_black)  % Handle "black" differently than other colors
                condition1 = 1;
                current_color = 2;
                break;
            elseif( a >= a_range(1,i) && a <= a_range(2,i) && b >= b_range(1,i) && b <= b_range(2,i) )
                condition1 = 1;
                current_color = i;
                break;
            end
            
        end
    end
    
    % Blob analysis
    if( condition1 == 1 )
        
        for i = 1:rows
            for j = 1:cols
                if(LabelMatrix(i,j) ~= k)
                    LogicMatrix(i,j) = false;
                else
                    LogicMatrix(i,j) = true;
                    bw_image(i,j) = 1;
                end
            end
        end

        [TArea,TCentroid,TBBox,TMajorAxis,TMinorAxis,TOrientation,TEccent,TExtent,TNumBlobs] = step(hblob,LogicMatrix);

        for i = 1:TNumBlobs
            if(blob_count + TNumBlobs <= max_num_blobs)

                blob_centroids(1,blob_count+i) = TCentroid(1,i);
                blob_centroids(2,blob_count+i) = TCentroid(2,i);

                ii = round(blob_centroids(1,blob_count+i));
                jj = round(blob_centroids(2,blob_count+i));

                blob_hues(1,blob_count+i) = ref_colors( LabelMatrix(ii,jj), 1 );
                blob_hues(2,blob_count+i) = ref_colors( LabelMatrix(ii,jj), 2 );
                blob_hues(3,blob_count+i) = ref_colors( LabelMatrix(ii,jj), 3 );

                blob_area(blob_count+i) = TArea(i);
                blob_bbox(blob_count+i) = TBBox(i);
                blob_major_axis(blob_count+i) = TMajorAxis(i);
                blob_minor_axis(blob_count+i) = TMinorAxis(i);
                blob_eccentricity(blob_count+i) = TEccent(i);
                blob_extent(blob_count+i) = TExtent(i);
                blob_orientation(blob_count+i) = TOrientation(i);
                
                blob_color(blob_count+i) = current_color;

            end
        end

        blob_count = blob_count + double(TNumBlobs);

    end
    
end


return

== matlab function Blob_Analysis/IterativeSegmentation/Low Pass Filter/Low Pass Filter ==
  data: I input double; Iout output double
function Iout = GaussianBlurr(I)
% This function calculates the gaussian blur of an intensity image

sigma = sqrt(2);

Grows = 3;    % Gaussian matrix rows
Gcols = 3;    % Gaussian matrix columns

[Irows Icols] = size(I);

Iout = double(zeros(Irows,Icols));

Trows = Irows - Grows + 1;
Tcols = Icols - Gcols + 1;
Itemp = double(zeros(Trows,Tcols));

G = zeros(Grows,Gcols);

FirstRow = ceil(-Grows/2);
LastRow = floor(Grows/2);
FirstCol = ceil(-Gcols/2);
LastCol = floor(Gcols/2);
Gsum = 0;
for i=FirstRow:LastRow
    for j = FirstCol:LastCol
        G(i-FirstRow+1,j-FirstCol+1) = exp(-(j*j+i*i)/(2*sigma*sigma));
        Gsum = Gsum + G(i-FirstRow+1,j-FirstCol+1);
    end
end

G = G./Gsum;

Itemp = conv2(double(I),double(G),'valid');

% reflect boundaries to keep image the same size
% top
Iout((1:LastRow),(LastCol+1:Icols-LastCol)) = Itemp((1:LastRow),(1:Tcols));
% bottom
Iout((Irows-LastRow+1:Irows),(LastCol+1:Icols-LastCol)) = Itemp((Trows-LastRow+1:Trows),(1:Tcols));
% left
Iout((1+LastRow:Irows-LastRow),(1:LastCol)) = Itemp((1:Trows),(1:LastCol));
% right
Iout((1+LastRow:Irows-LastRow),(Icols-LastCol+1:Icols)) = Itemp((1:Trows),(Tcols-LastCol+1:Tcols));
% center
Iout((1+LastRow:Irows-LastRow),(1+LastCol:Icols-LastCol)) = Itemp;
% top left corner
Iout(1:LastRow,1:LastCol) = Itemp(1:LastRow,1:LastCol);
% top right corner
Iout(1:LastRow,Icols-LastCol:Icols) = Itemp(1:LastRow,Tcols-LastCol:Tcols);
% bottom left corner
Iout(Irows-LastRow:Irows,1:LastCol) = Itemp(Trows-LastRow:Trows,1:LastCol);
% bottom right corner
Iout(Irows-LastRow:Irows,Icols-LastCol:Icols) = Itemp(Trows-LastRow:Trows,Tcols-LastCol:Tcols);

return

== matlab function Blob_Analysis/IterativeSegmentation/Low Pass Filter/Low Pass Filter1 ==
  data: I input double; Iout output double
function Iout = GaussianBlurr(I)
% This function calculates the gaussian blur of an intensity image

sigma = sqrt(2);

Grows = 3;    % Gaussian matrix rows
Gcols = 3;    % Gaussian matrix columns

[Irows Icols] = size(I);

Iout = double(zeros(Irows,Icols));

Trows = Irows - Grows + 1;
Tcols = Icols - Gcols + 1;
Itemp = double(zeros(Trows,Tcols));

G = zeros(Grows,Gcols);

FirstRow = ceil(-Grows/2);
LastRow = floor(Grows/2);
FirstCol = ceil(-Gcols/2);
LastCol = floor(Gcols/2);
Gsum = 0;
for i=FirstRow:LastRow
    for j = FirstCol:LastCol
        G(i-FirstRow+1,j-FirstCol+1) = exp(-(j*j+i*i)/(2*sigma*sigma));
        Gsum = Gsum + G(i-FirstRow+1,j-FirstCol+1);
    end
end

G = G./Gsum;

Itemp = conv2(double(I),double(G),'valid');

% reflect boundaries to keep image the same size
% top
Iout((1:LastRow),(LastCol+1:Icols-LastCol)) = Itemp((1:LastRow),(1:Tcols));
% bottom
Iout((Irows-LastRow+1:Irows),(LastCol+1:Icols-LastCol)) = Itemp((Trows-LastRow+1:Trows),(1:Tcols));
% left
Iout((1+LastRow:Irows-LastRow),(1:LastCol)) = Itemp((1:Trows),(1:LastCol));
% right
Iout((1+LastRow:Irows-LastRow),(Icols-LastCol+1:Icols)) = Itemp((1:Trows),(Tcols-LastCol+1:Tcols));
% center
Iout((1+LastRow:Irows-LastRow),(1+LastCol:Icols-LastCol)) = Itemp;
% top left corner
Iout(1:LastRow,1:LastCol) = Itemp(1:LastRow,1:LastCol);
% top right corner
Iout(1:LastRow,Icols-LastCol:Icols) = Itemp(1:LastRow,Tcols-LastCol:Tcols);
% bottom left corner
Iout(Irows-LastRow:Irows,1:LastCol) = Itemp(Trows-LastRow:Trows,1:LastCol);
% bottom right corner
Iout(Irows-LastRow:Irows,Icols-LastCol:Icols) = Itemp(Trows-LastRow:Trows,Tcols-LastCol:Tcols);

return
